simulink model "motor_pid_model_2018"  (R2017a)
settings: Solver=VariableStepAuto  StartTime=0.0  StopTime=1  FixedStep=1e-4  RelTol=1e-4
InitFcn:
  | Tw=0.01;     %Ancho de Ventana
  | ppv=20;      %Pulsos por vuelta
  | Ts=1e-4;     %Tiempo de muestreo
  | 
  | Kp=0.001;
  | Kd=0.02;
  | Ki=0.4;
  | h=Tw;
  | N=100;
  | 
  | % Los valores de num, den se obtienen de punto_2.m
  | % Fueron hardcodeados por comodidad.
  | 
  | num = [0 0.7770 0];
  | den = [1.0000 -0.9918 -0.0061];
settings Model: Creator=Martin  LastModifiedBy=Alan

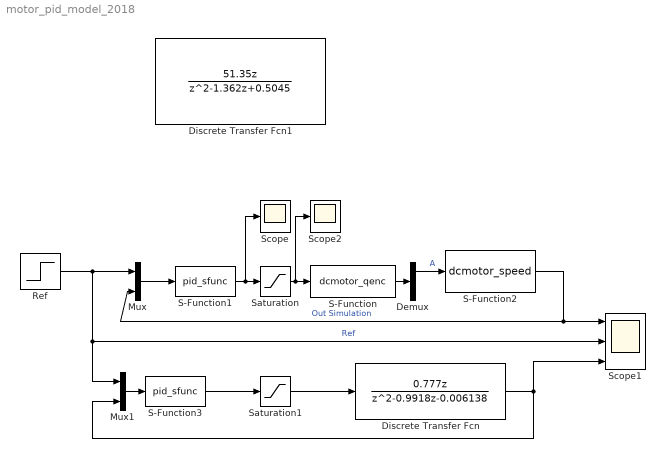
== system motor_pid_model_2018 ==
  Demux : Demux  Outputs=2
  Discrete Transfer Fcn : DiscreteTransferFcn  Numerator=[0.777 0]  Denominator=[1 -0.9918 -0.006138]  SampleTime=Ts
  Discrete Transfer Fcn1 : DiscreteTransferFcn  Numerator=[51.35 0]  Denominator=[1 -1.362 0.5045]  SampleTime=0.02
  Mux : Mux  Inputs=2
  Mux1 : Mux  Inputs=2
  Ref : Step  Time=0.2  After=4200  SampleTime=Ts
  S-Function : S-Function  FunctionName=dcmotor_qenc  Parameters=ppv  SFunctionDeploymentMode=off  EnableBusSupport=off
  S-Function1 : S-Function  FunctionName=pid_sfunc  Parameters=0.00266,0.000897,15.9,100,0.02  SFunctionDeploymentMode=off  EnableBusSupport=off
  S-Function2 : S-Function  FunctionName=dcmotor_speed  Parameters=Ts,ppv,Tw  SFunctionDeploymentMode=off  EnableBusSupport=off
  S-Function3 : S-Function  FunctionName=pid_sfunc  Parameters=0.00266,0.000897,15.9,100,0.02  SFunctionDeploymentMode=off  EnableBusSupport=off
  Saturation : Saturate  UpperLimit=30  LowerLimit=-30
  Saturation1 : Saturate  UpperLimit=30  LowerLimit=-30
  Scope : Scope
  Scope1 : Scope  NumInputPorts=3
  Scope2 : Scope
  wires:
  Ref/1 -> Mux/1, Scope1/2, Mux1/1  "Ref"
  S-Function/1 -> Demux/1
  Demux/1 -> S-Function2/1  "A"
  S-Function2/1 -> Scope1/1, Mux/2  "Out Simulation"
  Mux/1 -> S-Function1/1
  Saturation/1 -> Scope2/1, S-Function/1
  S-Function1/1 -> Scope/1, Saturation/1
  Mux1/1 -> S-Function3/1
  S-Function3/1 -> Saturation1/1
  Saturation1/1 -> Discrete Transfer Fcn/1
  Discrete Transfer Fcn/1 -> Mux1/2, Scope1/3
